simulink model "Boost_Converter"  (R2018b)
settings: Solver=VariableStepAuto  StartTime=0.0  StopTime=100  RelTol=1e-3
libraries: pePwmGenerator x1
settings Model: Creator=Vishant  LastModifiedBy=Vishant

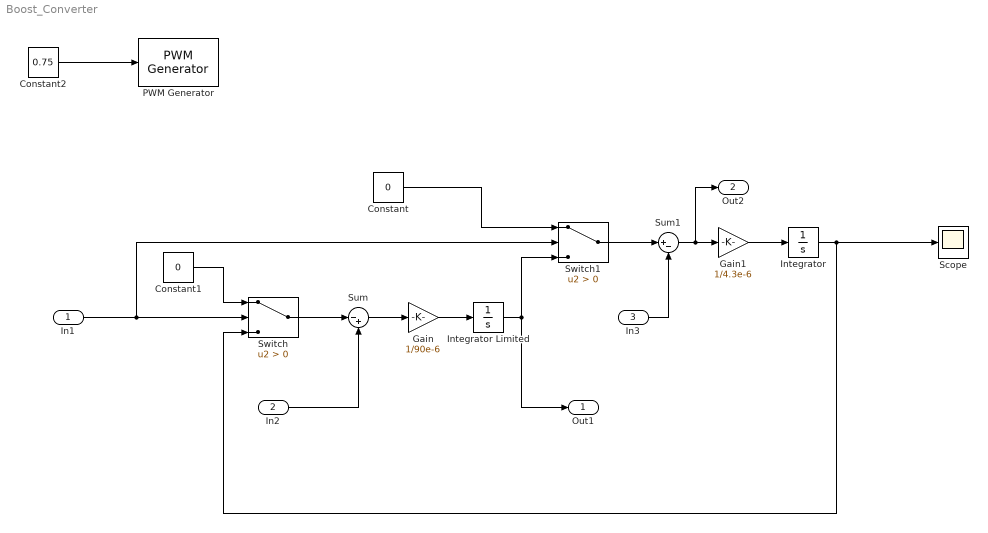
== system Boost_Converter ==
  In1 : Inport
  In2 : Inport  Port=2
  In3 : Inport  Port=3
  Constant : Constant  Value=0
  Constant1 : Constant  Value=0
  Constant2 : Constant  Value=0.75
  Gain : Gain  Gain=1/90e-6
  Gain1 : Gain  Gain=1/4.3e-6
  Integrator : Integrator
  Integrator Limited : Integrator  LimitOutput=on  UpperSaturationLimit=1  LowerSaturationLimit=0
  PWM Generator : pePwmGenerator/PWM Generator  CarrCount=Up  Tper=0.001  Ts=5e-5
  Scope : Scope
  Sum : Sum  Inputs=|-+
  Sum1 : Sum  Inputs=|+-
  Switch : Switch  Criteria=u2 > Threshold
  Switch1 : Switch  Criteria=u2 > Threshold
  Out1 : Outport
  Out2 : Outport  Port=2
  wires:
  Switch/1 -> Sum/1
  In2/1 -> Sum/2
  In1/1 -> Switch1/2, Switch/2
  Constant1/1 -> Switch/1
  Sum/1 -> Gain/1
  Gain/1 -> Integrator Limited/1
  Integrator Limited/1 -> Out1/1, Switch1/3
  Constant/1 -> Switch1/1
  Switch1/1 -> Sum1/1
  In3/1 -> Sum1/2
  Sum1/1 -> Out2/1, Gain1/1
  Gain1/1 -> Integrator/1
  Integrator/1 -> Scope/1, Switch/3
  Constant2/1 -> PWM Generator/1
